simulink model "PI_VC_vs_UPI_CC_3ph_4w_v2023b"  (R2023b)
settings: Solver=FixedStepDiscrete  StartTime=0.0  StopTime=14  FixedStep=Ts_Power  MaxStep=1e-4  RelTol=1e-3
InitFcn:
  | run PI_VC_vs_UPI_CC_ini;
values from neighbouring files (symbols this model uses):
  C = 4e-6    (= 4e-06)    [PI_OL_vs_PI_CC_ini.m]    (also in PI_VC_vs_UPI_CC_ini.m)
  C_2 = 4e-6    (= 4e-06)    [PI_OL_vs_PI_CC_ini.m]    (also in PI_VC_vs_UPI_CC_ini.m)
  K_i_pll = 1.8/0.00251    (= 717.131474104)    [PI_OL_vs_PI_CC_ini.m]    (also in PI_VC_vs_UPI_CC_ini.m)
  K_p_pll = 1.8    [PI_OL_vs_PI_CC_ini.m]    (also in PI_VC_vs_UPI_CC_ini.m)
  Kp_i = 1*(L_t2 + L_s2)/tau_i    (= 2.5)    [PI_OL_vs_PI_CC_ini.m]    (also in PI_VC_vs_UPI_CC_ini.m)
  Kr_i = 2*(R_t2 + R_s2)/tau_i    (= 157.079632679)    [PI_OL_vs_PI_CC_ini.m]    (also in PI_VC_vs_UPI_CC_ini.m)
  L_line_12_13 = X_line_12_13/(2*pi*50)    (= 0.000798957814321)    [PI_OL_vs_PI_CC_ini.m]    (also in PI_VC_vs_UPI_CC_ini.m)
  L_line_13_14 = X_line_13_14/(2*pi*50)    (= 0.000200535228296)    [PI_OL_vs_PI_CC_ini.m]    (also in PI_VC_vs_UPI_CC_ini.m)
  L_n = L_t2 + L_s2    (= 0.0025)    [PI_OL_vs_PI_CC_ini.m]    (also in PI_VC_vs_UPI_CC_ini.m)
  L_s = 1.25e-3    (= 0.00125)    [PI_OL_vs_PI_CC_ini.m]    (also in PI_VC_vs_UPI_CC_ini.m)
  L_s2 = 1.25e-3    (= 0.00125)    [PI_OL_vs_PI_CC_ini.m]    (also in PI_VC_vs_UPI_CC_ini.m)
  L_t = 1.25e-3    (= 0.00125)    [PI_OL_vs_PI_CC_ini.m]    (also in PI_VC_vs_UPI_CC_ini.m)
  L_t2 = 1.25e-3    (= 0.00125)    [PI_OL_vs_PI_CC_ini.m]    (also in PI_VC_vs_UPI_CC_ini.m)
  omega = 2*pi*f    (= 314.159265359)    [PI_OL_vs_PI_CC_ini.m]    (also in PI_VC_vs_UPI_CC_ini.m)
  params_pi_cc = [S_b,U_b,K_p,T_p,K_q,T_q,X,R]    [PI_OL_vs_PI_CC_ini.m]    (also in PI_VC_vs_UPI_CC_ini.m)
  params_pi_vc = [S_b,U_b,K_p,T_p,K_q,T_q,Xv,Rv]    [PI_OL_vs_PI_CC_ini.m]    (also in PI_VC_vs_UPI_CC_ini.m)
  params_vc_cc = [R_t;L_t;R_s;L_s;K_pi;K_ii;C;K_pv;K_iv]    [PI_OL_vs_PI_CC_ini.m]    (also in PI_VC_vs_UPI_CC_ini.m)
  R_d = 10    [PI_OL_vs_PI_CC_ini.m]    (also in PI_VC_vs_UPI_CC_ini.m)
  R_d2 = 10    [PI_OL_vs_PI_CC_ini.m]    (also in PI_VC_vs_UPI_CC_ini.m)
  R_line_12_13 = (0.06)*Length    (= 0.24)    [PI_OL_vs_PI_CC_ini.m]    (also in PI_VC_vs_UPI_CC_ini.m)
  R_line_13_14 = (0.025)*Length    (= 0.1)    [PI_OL_vs_PI_CC_ini.m]    (also in PI_VC_vs_UPI_CC_ini.m)
  R_n = L_n*omega/10    (= 0.0785398163397)    [PI_OL_vs_PI_CC_ini.m]    (also in PI_VC_vs_UPI_CC_ini.m)
  R_s = L_s*omega/10    (= 0.0392699081699)    [PI_OL_vs_PI_CC_ini.m]    (also in PI_VC_vs_UPI_CC_ini.m)
  R_s2 = L_s*omega/10    (= 0.0392699081699)    [PI_OL_vs_PI_CC_ini.m]    (also in PI_VC_vs_UPI_CC_ini.m)
  R_t = L_t*omega/10    (= 0.0392699081699)    [PI_OL_vs_PI_CC_ini.m]    (also in PI_VC_vs_UPI_CC_ini.m)
  R_t2 = L_t*omega/10    (= 0.0392699081699)    [PI_OL_vs_PI_CC_ini.m]    (also in PI_VC_vs_UPI_CC_ini.m)
  S_b = 20e3    (= 20000)    [PI_OL_vs_PI_CC_ini.m]    (also in PI_VC_vs_UPI_CC_ini.m)
  Ts_Control = 50e-6    (= 5e-05)    [PI_OL_vs_PI_CC_ini.m]    (also in PI_VC_vs_UPI_CC_ini.m)
  Ts_Power = 50e-6    (= 5e-05)    [PI_OL_vs_PI_CC_ini.m]    (also in PI_VC_vs_UPI_CC_ini.m)
  v_dc = 800    [PI_OL_vs_PI_CC_ini.m]    (also in PI_VC_vs_UPI_CC_ini.m)
undefined symbols (not defined in the file or in its folder): DiscIntNeverNeededParam, omega_ref
libraries: spsFirstOrderFilterLib x32, spsUniversalBridgeLib x10, spsThreePhaseSeriesRLCBranchLib x9, spsPowerLib x6, spsThreePhaseVIMeasurementLib x6, eeGeneralControl x5, spsSeriesRLCLoadLib x5, spsRMSLib x4, spsSeriesRLCBranchLib x4, spsPower3phInstantaneousLib x3, spsThreePhaseBreakerLib x3, spsDCVoltageSourceLib x2
(part 2 of 3)

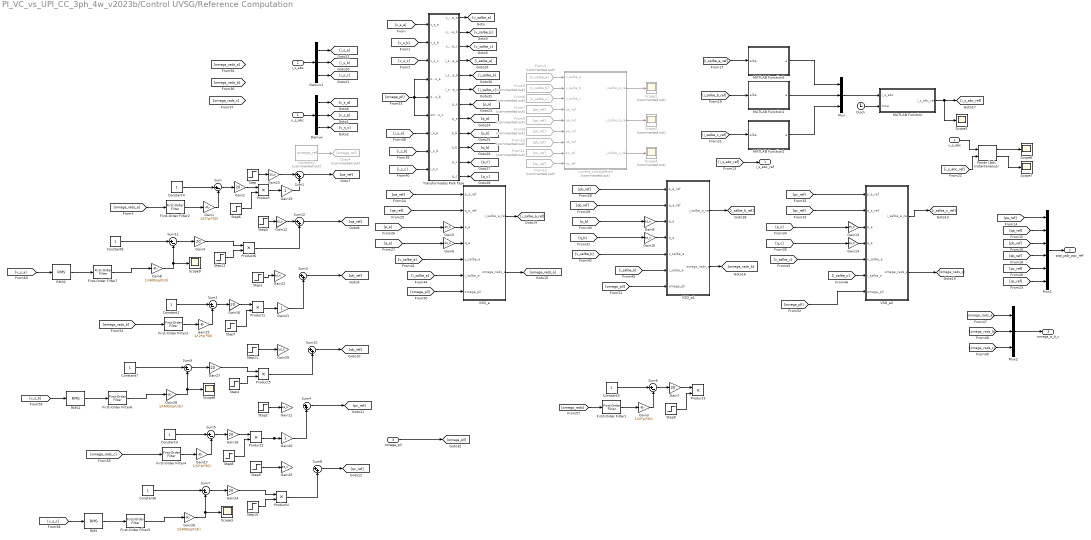
== system PI_VC_vs_UPI_CC_3ph_4w_v2023b/Control UVSG/Reference Computation ==
  v_s_abc : Inport
  i_s_abc : Inport  Port=2
  omega_pll : Inport  Port=3
  Clock : Clock
  Constant{1,3..8} (7 alike) : Constant
  Constant2 : Constant  Commented=on  Value=omega_ref
  Demux : Demux  Outputs=3
  Demux1 : Demux  Outputs=3
  First-Order Filter{1..7} (7 alike) : spsFirstOrderFilterLib/First-Order Filter  FilterType=Lowpass  Tc=10e-3  Ts=Ts_Control  Initialize=on  Vac_Init=[0, 0, 60]  Vdc_Init=0  PlotResponse=off  FreqRange="[0,  200,  1]"
  From10 : From  Commented=on  GotoTag=qb_ref
  From11 : From  Commented=on  GotoTag=pc_ref
  From12 : From  Commented=on  GotoTag=qc_ref
  From4 : From  Commented=on  GotoTag=v_salbe_a
  From5 : From  Commented=on  GotoTag=v_salbe_b
  From6 : From  Commented=on  GotoTag=v_salbe_c
  From7 : From  Commented=on  GotoTag=pa_ref
  From8 : From  Commented=on  GotoTag=pb_ref
  From9 : From  Commented=on  GotoTag=qa_ref
  Gain{1,3,15,17} (4 alike) : Gain  Gain=1/(2*pi*50)
  Gain{5..6,9..14,22..23,25,29} (12 alike) : Gain  Gain=3/S_b
  Gain{2,4,7,16,18,24,27} (7 alike) : Gain  Gain=20
  Gain19 : Gain
  Gain20 : Gain
  Gain21 : Gain
  Gain26 : Gain  Gain=1/(400/sqrt(3))
  Gain28 : Gain  Gain=1/(400/sqrt(3))
  Gain8 : Gain  Gain=1/(400/sqrt(3))
  Goto4 : Goto  Commented=on  GotoTag=omega_ref
  MATLAB Function : MATLAB Function  TreatAsAtomicUnit=on
  MATLAB Function1 : MATLAB Function  TreatAsAtomicUnit=on
  MATLAB Function2 : MATLAB Function  TreatAsAtomicUnit=on
  MATLAB Function5 : MATLAB Function  TreatAsAtomicUnit=on
  Mux : Mux  Inputs=3
  Mux1 : Mux  Inputs=6
  Mux2 : Mux  Inputs=3
  "Power (3ph, Instantaneous)" : spsPower3phInstantaneousLib/Power (3ph, Instantaneous)
  Product{,1..6} (7 alike) : Product
  RMS : spsRMSLib/RMS  TrueRMS=on  Freq=50  RMSInit=230  Ts=Ts_Control
  RMS1 : spsRMSLib/RMS  TrueRMS=on  Freq=50  RMSInit=230  Ts=Ts_Control
  RMS2 : spsRMSLib/RMS  TrueRMS=on  Freq=50  RMSInit=230  Ts=Ts_Control
  Scope1 : Scope  Commented=on
  Scope2 : Scope  Commented=on
  Scope{3,5..9} (6 alike) : Scope
  Scope4 : Scope  Commented=on
  Step : Step  Time=11  After=1000  SampleTime=0
  Step1 : Step  Time=6  After=1000  SampleTime=0
  Step{4,6..8,10,12} (6 alike) : Step  Time=7  SampleTime=0
  Step11 : Step  Time=0  After=0  SampleTime=0
  Step2 : Step  Time=6  After=1000  SampleTime=0
  Step3 : Step  Time=11  After=1000  SampleTime=0
  Step5 : Step  Time=0  After=0  SampleTime=0
  Step9 : Step  SampleTime=0
  Sum{,2,5..7,9,11} (7 alike) : Sum  Inputs=|+-
  Sum{1,3..4,8,10,12} (6 alike) : Sum  Inputs=|++
  Transformadas Park fase : Subsystem
  VSG_a : Subsystem
  VSG_a1 : Subsystem
  VSG_a2 : Subsystem
  current_computation : MATLAB Function  Commented=on  TreatAsAtomicUnit=on
  "v_s_abc " : InportShadow
  i_s_abc_ref : Outport  VectorParamsAs1DForOutWhenUnconnected=off
  pqa_pqb_pqc_ref : Outport  Port=2  VectorParamsAs1DForOutWhenUnconnected=off
  omega_a_b_c : Outport  Port=3  VectorParamsAs1DForOutWhenUnconnected=off
  wires:
  v_s_abc/1 -> Demux/1
  Demux/1 -> [v_s_a]
  Demux/2 -> [v_s_b]
  Demux/3 -> [v_s_c]
  Constant2/1 -> Goto4/1
  [v_s_a] -> Transformadas Park fase/1(v_s_a)
  [v_s_b] -> Transformadas Park fase/2(v_s_b)
  [v_s_c] -> Transformadas Park fase/3(v_s_c)
  Transformadas Park fase/1(v_salbe_a) -> [v_salbe_a]
  Transformadas Park fase/3(v_salbe_c) -> [v_salbe_c]
  Transformadas Park fase/2(v_salbe_b) -> [v_salbe_b]
  From4/1 -> current_computation/1(v_salbe_a)
  From5/1 -> current_computation/2(v_salbe_b)
  From6/1 -> current_computation/3(v_salbe_c)
  From7/1 -> current_computation/4(pa_ref)
  From9/1 -> current_computation/5(qa_ref)
  From8/1 -> current_computation/6(pb_ref)
  From10/1 -> current_computation/7(qb_ref)
  From11/1 -> current_computation/8(pc_ref)
  From12/1 -> current_computation/9(qc_ref)
  current_computation/1(i_salbe_a_ref) -> Scope1/1
  current_computation/2(i_salbe_b_ref) -> Scope2/1
  current_computation/3(i_salbe_c_ref) -> Scope4/1
  [i_salbe_b_ref] -> MATLAB Function1/1(albe)
  [i_salbe_c_ref] -> MATLAB Function2/1(albe)
  MATLAB Function5/1(a) -> Mux/1
  [i_s_abc_ref] -> "Power (3ph, Instantaneous)"/2
  "v_s_abc "/1 -> "Power (3ph, Instantaneous)"/1
  "Power (3ph, Instantaneous)"/1 -> Scope6/1
  "Power (3ph, Instantaneous)"/2 -> Scope7/1
  [i_s_abc_ref] -> i_s_abc_ref/1
  [i_salbe_a_ref] -> MATLAB Function5/1(albe)
  MATLAB Function1/1(a) -> Mux/2
  MATLAB Function2/1(a) -> Mux/3
  [pa_ref] -> Mux1/1
  [qa_ref] -> Mux1/2
  [pb_ref] -> Mux1/3
  [qb_ref] -> Mux1/4
  [pc_ref] -> Mux1/5
  [qc_ref] -> Mux1/6
  Mux1/1 -> pqa_pqb_pqc_ref/1
  VSG_a/2(omega_rads_a) -> [omega_rads_a]
  VSG_a1/2(omega_rads_a) -> [omega_rads_b]
  Demux1/3 -> [i_s_c]
  Demux1/2 -> [i_s_b]
  Demux1/1 -> [i_s_a]
  i_s_abc/1 -> Demux1/1
  [i_s_a] -> Transformadas Park fase/7(i_s_a)
  [i_s_b] -> Transformadas Park fase/8(i_s_b)
  [i_s_c] -> Transformadas Park fase/9(i_s_c)
  Transformadas Park fase/7(p_a) -> [p_a]
  Transformadas Park fase/8(q_a) -> [q_a]
  Transformadas Park fase/9(p_b) -> [p_b]
  Transformadas Park fase/10(q_b) -> [q_b]
  Transformadas Park fase/11(p_c) -> [p_c]
  Transformadas Park fase/12(q_c) -> [q_c]
  Transformadas Park fase/4(i_salbe_a) -> [i_salbe_a]
  Transformadas Park fase/5(i_salbe_b) -> [i_salbe_b]
  Transformadas Park fase/6(i_salbe_c) -> [i_salbe_c]
  VSG_a/1(i_salbe_a_ref) -> [i_salbe_a_ref]
  VSG_a1/1(i_salbe_a_ref) -> [i_salbe_b_ref]
  VSG_a2/1(i_salbe_a_ref) -> [i_salbe_c_ref]
  [pa_ref] -> VSG_a/1(p_a_ref)
  [qa_ref] -> VSG_a/2(q_a_ref)
  Gain5/1 -> VSG_a/3(p_a)
  Gain6/1 -> VSG_a/4(q_a)
  [pb_ref] -> VSG_a1/1(p_a_ref)
  [qb_ref] -> VSG_a1/2(q_a_ref)
  Gain9/1 -> VSG_a1/3(p_a)
  Gain10/1 -> VSG_a1/4(q_a)
  [qc_ref] -> VSG_a2/2(q_a_ref)
  Gain13/1 -> VSG_a2/3(p_a)
  Gain14/1 -> VSG_a2/4(q_a)
  [p_a] -> Gain5/1
  [q_a] -> Gain6/1
  [q_b] -> Gain10/1
  [p_c] -> Gain13/1
  [q_c] -> Gain14/1
  VSG_a2/2(omega_rads_a) -> [omega_rads_c]
  [v_salbe_a] -> VSG_a/5(v_salbe_a)
  [v_salbe_b] -> VSG_a1/5(v_salbe_a)
  [v_salbe_c] -> VSG_a2/5(v_salbe_a)
  [p_b] -> Gain9/1
  [i_salbe_a] -> VSG_a/6(i_salbe_a)
  [i_salbe_b] -> VSG_a1/6(i_salbe_a)
  [i_salbe_c] -> VSG_a2/6(i_salbe_a)
  Mux2/1 -> omega_a_b_c/1
  [omega_rads_a] -> Mux2/1
  [omega_rads_b] -> Mux2/2
  [omega_rads_c] -> Mux2/3
  omega_pll/1 -> [omega_pll]
  [omega_pll] -> VSG_a/7(omega_pll)
  [omega_pll] -> VSG_a1/7(omega_pll)
  [omega_pll] -> VSG_a2/7(omega_pll)
  Mux/1 -> MATLAB Function/1(i_s_abc)
  MATLAB Function/1(i_s_abc_ref) -> Scope5/1, [i_s_abc_ref]
  Clock/1 -> MATLAB Function/2(time)
  Gain2/1 -> Product/1
  [omega_rads_a] -> First-Order Filter2/1
  Step6/1 -> Product/2
  Gain1/1 -> Sum/2
  Constant4/1 -> Sum/1
  Sum/1 -> Gain2/1
  Product/1 -> Gain19/1
  Product1/1 -> Gain21/1
  Sum2/1 -> Gain16/1
  Constant1/1 -> Sum2/1
  Gain15/1 -> Sum2/2
  Step7/1 -> Product1/2
  [omega_rads_b] -> First-Order Filter3/1
  Gain16/1 -> Product1/1
  Gain18/1 -> Product2/1
  [omega_rads_c] -> First-Order Filter4/1
  Step8/1 -> Product2/2
  Gain17/1 -> Sum5/2
  Constant3/1 -> Sum5/1
  Sum5/1 -> Gain18/1
  Sum1/1 -> [pa_ref]
  Sum3/1 -> [pb_ref]
  Product2/1 -> Gain20/1
  Sum4/1 -> [pc_ref]
  Step2/1 -> Gain11/1
  Step1/1 -> Gain22/1
  Step/1 -> Gain23/1
  [pc_ref] -> VSG_a2/1(p_a_ref)
  [omega_pll] -> Transformadas Park fase/6(omega_rads_c), Transformadas Park fase/4(omega_rads_a), Transformadas Park fase/5(omega_rads_b)
  First-Order Filter1/1 -> Gain3/1
  [omega_rads] -> First-Order Filter1/1
  Step9/1 -> Product3/2
  Gain7/1 -> Product3/1
  Sum6/1 -> Gain7/1
  Gain3/1 -> Sum6/2
  Constant5/1 -> Sum6/1
  First-Order Filter2/1 -> Gain1/1
  First-Order Filter3/1 -> Gain15/1
  First-Order Filter4/1 -> Gain17/1
  Gain19/1 -> Sum1/2
  Gain21/1 -> Sum3/2
  Gain20/1 -> Sum4/2
  Gain23/1 -> Sum1/1
  Step5/1 -> Gain25/1
  Step10/1 -> Product4/2
  Gain24/1 -> Product4/1
  Sum7/1 -> Gain24/1
  Gain26/1 -> Scope3/1, Sum7/2
  [v_s_c] -> RMS/1
  Constant6/1 -> Sum7/1
  RMS/1 -> First-Order Filter5/1
  Sum8/1 -> [qc_ref]
  Product4/1 -> Sum8/2
  RMS1/1 -> First-Order Filter6/1
  Constant7/1 -> Sum9/1
  [v_s_b] -> RMS1/1
  Gain28/1 -> Sum9/2, Scope8/1
  Sum9/1 -> Gain27/1
  Gain27/1 -> Product5/1
  Step4/1 -> Product5/2
  Sum10/1 -> [qb_ref]
  Product5/1 -> Sum10/2
  Step11/1 -> Gain29/1
  Product6/1 -> Sum12/2
  Sum11/1 -> Gain4/1
  Gain4/1 -> Product6/1
  RMS2/1 -> First-Order Filter7/1
  [v_s_a] -> RMS2/1
  Gain8/1 -> Sum11/2, Scope9/1
  Step12/1 -> Product6/2
  Constant8/1 -> Sum11/1
  Gain12/1 -> Sum12/1
  Step3/1 -> Gain12/1
  Sum12/1 -> [qa_ref]
  First-Order Filter7/1 -> Gain8/1
  First-Order Filter6/1 -> Gain28/1
  First-Order Filter5/1 -> Gain26/1

== system PI_VC_vs_UPI_CC_3ph_4w_v2023b/Plant/Subsystem2 ==
  eta_abc : Inport
  eta_n : Inport  Port=2
  DC Voltage Source : spsDCVoltageSourceLib/DC Voltage Source  Amplitude=v_dc  Measurements=None
  Demux : Demux  Outputs=3
  Series RLC Branch : spsSeriesRLCBranchLib/Series RLC Branch  LConnTagsString=__new0  RConnTagsString=__new0  BranchType=RL  Resistance=R_n  Inductance=L_n  SetiL0=off  InitialCurrent=0  Capacitance=1e-6  Setx0=off  InitialVoltage=0  Measurements=None
  Three-Phase Series RLC Branch : spsThreePhaseSeriesRLCBranchLib/Three-Phase Series RLC Branch  LConnTagsString=A|B|C  RConnTagsString=A|B|C  BranchType=RL  Resistance=R_t  Inductance=L_t  Capacitance=1e-6  Measurements=None
  Three-Phase Series RLC Branch1 : spsThreePhaseSeriesRLCBranchLib/Three-Phase Series RLC Branch  LConnTagsString=A|B|C  RConnTagsString=A|B|C  BranchType=RL  Resistance=R_s  Inductance=L_s  Capacitance=1e-6  Measurements=None
  Three-Phase Series RLC Branch2 : spsThreePhaseSeriesRLCBranchLib/Three-Phase Series RLC Branch  LConnTagsString=A|B|C  RConnTagsString=A|B|C  BranchType=RC  Resistance=R_d  Inductance=L_t  Capacitance=C  Measurements=None
  Three-Phase V-I Measurement : spsThreePhaseVIMeasurementLib/Three-Phase V-I Measurement  VoltageMeasurement=phase-to-ground  SetLabelV=off  LabelV=Vabc  Vpu=off  VpuLL=off  CurrentMeasurement=yes  SetLabelI=off  LabelI=Iabc  Ipu=off  Pbase=100e6  Vbase=500e3  OutputType=Complex  PhasorSimulation=off  PSBequivalent=0
  Three-Phase V-I Measurement2 : spsThreePhaseVIMeasurementLib/Three-Phase V-I Measurement  VoltageMeasurement=phase-to-ground  SetLabelV=off  LabelV=Vabc  Vpu=off  VpuLL=off  CurrentMeasurement=no  SetLabelI=off  LabelI=Iabc  Ipu=off  Pbase=100e6  Vbase=500e3  OutputType=Complex  PhasorSimulation=off  PSBequivalent=0
  Universal Bridge : spsUniversalBridgeLib/Universal Bridge  Commented=on  Arms=3  SnubberResistance=1e5  SnubberCapacitance=inf  Device=Average-model based VSC  Ron=1e-3  Lon=0  ForwardVoltages="[  0  0  ]"  ForwardVoltage=0  GTOparameters=[ 10e-6 , 20e-6 ]  IGBTparameters=[ 1e-6 , 2e-6 ]  Measurements=None  Measurements_2=None  converterType=Rectifier
  Universal Bridge{1..2,4..5} (4 alike) : spsUniversalBridgeLib/Universal Bridge  Arms=1  SnubberResistance=1e5  SnubberCapacitance=inf  Device=Average-model based VSC  Ron=1e-3  Lon=0  ForwardVoltages="[  0  0  ]"  ForwardVoltage=0  GTOparameters=[ 10e-6 , 20e-6 ]  IGBTparameters=[ 1e-6 , 2e-6 ]  Measurements=None  Measurements_2=None  converterType=Rectifier
  Voltage Measurement : spsVoltageMeasurementLib/Voltage Measurement  PhasorSimulation=off  OutputType=Complex  PSBequivalent=0
  a : PMIOPort  Side=Right
  b : PMIOPort  Port=2  Side=Right
  c : PMIOPort  Port=3  Side=Right
  n : PMIOPort  Port=4  Side=Right
  v_cabc : Outport
  i_tabc : Outport  Port=2
  v_tabc : Outport  Port=3
  v_dc : Outport  Port=4
  wires:
  Three-Phase V-I Measurement/2 -> i_tabc/1
  Three-Phase V-I Measurement2/1 -> v_cabc/1
  Three-Phase V-I Measurement/1 -> v_tabc/1
  eta_abc/1 -> Demux/1
  Voltage Measurement/1 -> v_dc/1
  Demux/1 -> Universal Bridge2/1
  Demux/2 -> Universal Bridge4/1
  Demux/3 -> Universal Bridge5/1
  eta_n/1 -> Universal Bridge1/1
  connections:
  Three-Phase V-I Measurement/RConn3 -- Three-Phase Series RLC Branch/LConn3
  Three-Phase V-I Measurement/LConn2 -- Universal Bridge4/LConn1
  Three-Phase V-I Measurement/RConn1 -- Three-Phase Series RLC Branch/LConn1
  Three-Phase V-I Measurement2/LConn3 -- Three-Phase Series RLC Branch/RConn3 -- Three-Phase Series RLC Branch1/LConn3
  DC Voltage Source/RConn1 -- Universal Bridge1/RConn1 -- Universal Bridge5/RConn1 -- Universal Bridge4/RConn1 -- Universal Bridge2/RConn1 -- Voltage Measurement/LConn1
  DC Voltage Source/LConn1 -- Universal Bridge1/RConn2 -- Universal Bridge2/RConn2 -- Universal Bridge4/RConn2 -- Universal Bridge5/RConn2 -- Voltage Measurement/LConn2
  Three-Phase Series RLC Branch2/LConn2 -- Three-Phase V-I Measurement2/RConn2
  Three-Phase Series RLC Branch2/LConn1 -- Three-Phase V-I Measurement2/RConn3
  Three-Phase Series RLC Branch1/LConn2 -- Three-Phase V-I Measurement2/LConn2 -- Three-Phase Series RLC Branch/RConn2
  Three-Phase Series RLC Branch/LConn2 -- Three-Phase V-I Measurement/RConn2
  Three-Phase V-I Measurement/LConn1 -- Universal Bridge2/LConn1
  Three-Phase Series RLC Branch1/LConn1 -- Three-Phase V-I Measurement2/LConn1 -- Three-Phase Series RLC Branch/RConn1
  Three-Phase V-I Measurement2/RConn1 -- Three-Phase Series RLC Branch2/LConn3
  Three-Phase Series RLC Branch2/RConn3 -- n/RConn1 -- Series RLC Branch/RConn1 -- Three-Phase Series RLC Branch2/RConn1 -- Three-Phase Series RLC Branch2/RConn2
  Three-Phase V-I Measurement/LConn3 -- Universal Bridge5/LConn1
  a/RConn1 -- Three-Phase Series RLC Branch1/RConn1
  b/RConn1 -- Three-Phase Series RLC Branch1/RConn2
  Three-Phase Series RLC Branch1/RConn3 -- c/RConn1
  Universal Bridge1/LConn1 -- Series RLC Branch/LConn1

== system PI_VC_vs_UPI_CC_3ph_4w_v2023b/Plant/Subsystem3 ==
  eta_abc : Inport
  eta_n : Inport  Port=2
  DC Voltage Source : spsDCVoltageSourceLib/DC Voltage Source  Amplitude=v_dc  Measurements=None
  Demux : Demux  Outputs=3
  Series RLC Branch : spsSeriesRLCBranchLib/Series RLC Branch  LConnTagsString=__new0  RConnTagsString=__new0  BranchType=RL  Resistance=R_n  Inductance=L_n  SetiL0=off  InitialCurrent=0  Capacitance=1e-6  Setx0=off  InitialVoltage=0  Measurements=None
  Three-Phase Series RLC Branch : spsThreePhaseSeriesRLCBranchLib/Three-Phase Series RLC Branch  LConnTagsString=A|B|C  RConnTagsString=A|B|C  BranchType=RL  Resistance=R_t2  Inductance=L_t2  Capacitance=1e-6  Measurements=None
  Three-Phase Series RLC Branch1 : spsThreePhaseSeriesRLCBranchLib/Three-Phase Series RLC Branch  LConnTagsString=A|B|C  RConnTagsString=A|B|C  BranchType=RL  Resistance=R_s2  Inductance=L_s2  Capacitance=1e-6  Measurements=None
  Three-Phase Series RLC Branch2 : spsThreePhaseSeriesRLCBranchLib/Three-Phase Series RLC Branch  LConnTagsString=A|B|C  RConnTagsString=A|B|C  BranchType=RC  Resistance=R_d2  Inductance=L_t  Capacitance=C_2  Measurements=None
  Three-Phase V-I Measurement : spsThreePhaseVIMeasurementLib/Three-Phase V-I Measurement  VoltageMeasurement=phase-to-ground  SetLabelV=off  LabelV=Vabc  Vpu=off  VpuLL=off  CurrentMeasurement=yes  SetLabelI=off  LabelI=Iabc  Ipu=off  Pbase=100e6  Vbase=500e3  OutputType=Complex  PhasorSimulation=off  PSBequivalent=0
  Three-Phase V-I Measurement2 : spsThreePhaseVIMeasurementLib/Three-Phase V-I Measurement  VoltageMeasurement=phase-to-ground  SetLabelV=off  LabelV=Vabc  Vpu=off  VpuLL=off  CurrentMeasurement=no  SetLabelI=off  LabelI=Iabc  Ipu=off  Pbase=100e6  Vbase=500e3  OutputType=Complex  PhasorSimulation=off  PSBequivalent=0
  Universal Bridge : spsUniversalBridgeLib/Universal Bridge  Commented=on  Arms=3  SnubberResistance=1e5  SnubberCapacitance=inf  Device=Average-model based VSC  Ron=1e-3  Lon=0  ForwardVoltages="[  0  0  ]"  ForwardVoltage=0  GTOparameters=[ 10e-6 , 20e-6 ]  IGBTparameters=[ 1e-6 , 2e-6 ]  Measurements=None  Measurements_2=None  converterType=Rectifier
  Universal Bridge{1..2,4..5} (4 alike) : spsUniversalBridgeLib/Universal Bridge  Arms=1  SnubberResistance=1e5  SnubberCapacitance=inf  Device=Average-model based VSC  Ron=1e-3  Lon=0  ForwardVoltages="[  0  0  ]"  ForwardVoltage=0  GTOparameters=[ 10e-6 , 20e-6 ]  IGBTparameters=[ 1e-6 , 2e-6 ]  Measurements=None  Measurements_2=None  converterType=Rectifier
  Voltage Measurement : spsVoltageMeasurementLib/Voltage Measurement  PhasorSimulation=off  OutputType=Complex  PSBequivalent=0
  a : PMIOPort  Side=Right
  b : PMIOPort  Port=2  Side=Right
  c : PMIOPort  Port=3  Side=Right
  n : PMIOPort  Port=4  Side=Right
  v_cabc : Outport
  i_tabc : Outport  Port=2
  v_tabc : Outport  Port=3
  v_dc : Outport  Port=4
  wires:
  eta_n/1 -> Universal Bridge1/1
  Demux/3 -> Universal Bridge5/1
  Demux/2 -> Universal Bridge4/1
  Demux/1 -> Universal Bridge2/1
  Voltage Measurement/1 -> v_dc/1
  eta_abc/1 -> Demux/1
  Three-Phase V-I Measurement/1 -> v_tabc/1
  Three-Phase V-I Measurement2/1 -> v_cabc/1
  Three-Phase V-I Measurement/2 -> i_tabc/1
  connections:
  Universal Bridge1/LConn1 -- Series RLC Branch/LConn1
  Three-Phase Series RLC Branch1/RConn3 -- c/RConn1
  b/RConn1 -- Three-Phase Series RLC Branch1/RConn2
  a/RConn1 -- Three-Phase Series RLC Branch1/RConn1
  Three-Phase V-I Measurement/LConn3 -- Universal Bridge5/LConn1
  n/RConn1 -- Three-Phase Series RLC Branch2/RConn2 -- Three-Phase Series RLC Branch2/RConn1 -- Series RLC Branch/RConn1 -- Three-Phase Series RLC Branch2/RConn3
  Three-Phase V-I Measurement2/RConn1 -- Three-Phase Series RLC Branch2/LConn3
  Three-Phase Series RLC Branch/RConn1 -- Three-Phase V-I Measurement2/LConn1 -- Three-Phase Series RLC Branch1/LConn1
  Three-Phase V-I Measurement/LConn1 -- Universal Bridge2/LConn1
  Three-Phase Series RLC Branch/LConn2 -- Three-Phase V-I Measurement/RConn2
  Three-Phase Series RLC Branch/RConn2 -- Three-Phase V-I Measurement2/LConn2 -- Three-Phase Series RLC Branch1/LConn2
  Three-Phase Series RLC Branch2/LConn1 -- Three-Phase V-I Measurement2/RConn3
  Three-Phase Series RLC Branch2/LConn2 -- Three-Phase V-I Measurement2/RConn2
  Universal Bridge1/RConn2 -- Universal Bridge5/RConn2 -- Universal Bridge4/RConn2 -- Universal Bridge2/RConn2 -- Voltage Measurement/LConn2 -- DC Voltage Source/LConn1
  Universal Bridge1/RConn1 -- Universal Bridge5/RConn1 -- Universal Bridge4/RConn1 -- Voltage Measurement/LConn1 -- DC Voltage Source/RConn1 -- Universal Bridge2/RConn1
  Three-Phase Series RLC Branch1/LConn3 -- Three-Phase Series RLC Branch/RConn3 -- Three-Phase V-I Measurement2/LConn3
  Three-Phase V-I Measurement/RConn1 -- Three-Phase Series RLC Branch/LConn1
  Three-Phase V-I Measurement/LConn2 -- Universal Bridge4/LConn1
  Three-Phase V-I Measurement/RConn3 -- Three-Phase Series RLC Branch/LConn3

== system PI_VC_vs_UPI_CC_3ph_4w_v2023b/Control UVSG/Control corriente en alpha-beta/Resonant Controller. Double Integrator ==
  i_sal_ref : Inport
  i_sal : Inport  Port=2
  Vdc : Inport  Port=3
  i_sbe_ref : Inport  Port=4
  i_sbe : Inport  Port=5
  omega_PLL : Inport  Port=6
  v_sal : Inport  Port=7
  v_sbe : Inport  Port=8
  Divide : Product  Inputs=*/
  Divide1 : Product  Inputs=*/
  Gain1 : Gain  Gain=Kp_i
  Gain10 : Gain  Gain=2
  Gain7 : Gain  Gain=2
  Gain8 : Gain  Gain=Kp_i
  Mux : Mux  Inputs=2
  Scope7 : Scope
  Subsystem1 : Subsystem
  Subsystem2 : Subsystem
  Sum{4..6,13} (4 alike) : Sum  Inputs=|++
  Sum7 : Sum  Inputs=|+-
  Sum9 : Sum  Inputs=|+-
  omega_PLL_1 : InportShadow  Port=6
  eta_albe : Outport
  wires:
  Gain1/1 -> Sum6/1
  Gain8/1 -> Sum13/1
  i_sbe_ref/1 -> Sum9/1
  omega_PLL_1/1 -> Subsystem1/2(omega_PLL)
  i_sal_ref/1 -> Sum7/1
  Sum13/1 -> Sum4/1
  Vdc/1 -> Divide/2, Divide1/2
  Sum5/1 -> Gain10/1
  Sum7/1 -> Subsystem1/1(error), Gain8/1, Scope7/1
  Sum6/1 -> Sum5/1
  Sum4/1 -> Gain7/1
  Divide1/1 -> Mux/2
  Divide/1 -> Mux/1
  Gain7/1 -> Divide/1
  Subsystem1/1(out) -> Sum13/2
  Sum9/1 -> Subsystem2/1(error), Gain1/1
  Subsystem2/1(out) -> Sum6/2
  v_sal/1 -> Sum4/2
  Gain10/1 -> Divide1/1
  omega_PLL/1 -> Subsystem2/2(omega_PLL)
  Mux/1 -> eta_albe/1
  i_sal/1 -> Sum7/2
  i_sbe/1 -> Sum9/2
  v_sbe/1 -> Sum5/2

== system PI_VC_vs_UPI_CC_3ph_4w_v2023b/Control UVSG/Control corriente en alpha-beta/Resonant Controller. Impulse invariant ==
  i_sal_ref : Inport
  i_sal : Inport  Port=2
  Vdc : Inport  Port=3
  i_sbe_ref : Inport  Port=4
  i_sbe : Inport  Port=5
  omega_PLL : Inport  Port=6
  v_sal : Inport  Port=7
  v_sbe : Inport  Port=8
  Divide : Product  Inputs=*/
  Divide1 : Product  Inputs=*/
  Gain1 : Gain  Gain=Kp_i
  Gain10 : Gain  Gain=2
  Gain7 : Gain  Gain=2
  Gain8 : Gain  Gain=Kp_i
  Mux : Mux  Inputs=2
  Scope7 : Scope
  Subsystem : Subsystem
  Subsystem1 : Subsystem
  Sum{4..6,13} (4 alike) : Sum  Inputs=|++
  Sum7 : Sum  Inputs=|+-
  Sum9 : Sum  Inputs=|+-
  omega_PLL_1 : InportShadow  Port=6
  eta_albe : Outport
  wires:
  Gain1/1 -> Sum6/1
  Gain8/1 -> Sum13/1
  i_sbe_ref/1 -> Sum9/1
  i_sal_ref/1 -> Sum7/1
  Sum13/1 -> Sum4/1
  Vdc/1 -> Divide/2, Divide1/2
  Sum5/1 -> Gain10/1
  Sum7/1 -> Subsystem1/1(error), Gain8/1, Scope7/1
  Sum6/1 -> Sum5/1
  Sum4/1 -> Gain7/1
  Divide1/1 -> Mux/2
  Divide/1 -> Mux/1
  Gain7/1 -> Divide/1
  Sum9/1 -> Subsystem/1(error), Gain1/1
  v_sal/1 -> Sum4/2
  Gain10/1 -> Divide1/1
  Mux/1 -> eta_albe/1
  i_sal/1 -> Sum7/2
  i_sbe/1 -> Sum9/2
  v_sbe/1 -> Sum5/2
  omega_PLL/1 -> Subsystem/2(omega_PLL)
  omega_PLL_1/1 -> Subsystem1/2(omega_PLL)
  Subsystem1/1(y) -> Sum13/2
  Subsystem/1(y) -> Sum6/2

== system PI_VC_vs_UPI_CC_3ph_4w_v2023b/Control UVSG/Control corriente en alpha-beta/Subsystem ==
  In1 : Inport
  Demux : Demux  Outputs=2
  Mux : Mux  Inputs=2
  Unit Delay1 : UnitDelay  SampleTime=Ts_Control  HasFrameUpgradeWarning=on
  Unit Delay2 : UnitDelay  SampleTime=Ts_Control  HasFrameUpgradeWarning=on
  Out1 : Outport
  wires:
  In1/1 -> Demux/1
  Demux/1 -> Unit Delay2/1
  Demux/2 -> Unit Delay1/1
  Mux/1 -> Out1/1
  Unit Delay2/1 -> Mux/1
  Unit Delay1/1 -> Mux/2

== system PI_VC_vs_UPI_CC_3ph_4w_v2023b/Control UVSG/Control corriente en alpha-beta/Subsystem1 ==
  In1 : Inport
  Demux : Demux  Outputs=2
  Mux : Mux  Inputs=2
  Unit Delay1 : UnitDelay  SampleTime=Ts_Control  HasFrameUpgradeWarning=on
  Unit Delay2 : UnitDelay  SampleTime=Ts_Control  HasFrameUpgradeWarning=on
  u_aux_1 : Outport
  wires:
  Unit Delay1/1 -> Mux/2
  Unit Delay2/1 -> Mux/1
  Mux/1 -> u_aux_1/1
  Demux/2 -> Unit Delay1/1
  Demux/1 -> Unit Delay2/1
  In1/1 -> Demux/1

== system PI_VC_vs_UPI_CC_3ph_4w_v2023b/Control UVSG/Control corriente en alpha-beta/Subsystem2 ==
  In1 : Inport
  Demux : Demux  Outputs=2
  Mux : Mux  Inputs=2
  Unit Delay1 : UnitDelay  SampleTime=Ts_Control  HasFrameUpgradeWarning=on
  Unit Delay2 : UnitDelay  SampleTime=Ts_Control  HasFrameUpgradeWarning=on
  Out1 : Outport
  wires:
  In1/1 -> Demux/1
  Demux/1 -> Unit Delay2/1
  Demux/2 -> Unit Delay1/1
  Mux/1 -> Out1/1
  Unit Delay2/1 -> Mux/1
  Unit Delay1/1 -> Mux/2

== system PI_VC_vs_UPI_CC_3ph_4w_v2023b/Control UVSG/Control corriente en alpha-beta/Subsystem3 ==
  In1 : Inport
  Demux : Demux  Outputs=2
  Mux : Mux  Inputs=2
  Unit Delay1 : UnitDelay  SampleTime=Ts_Control  HasFrameUpgradeWarning=on
  Unit Delay2 : UnitDelay  SampleTime=Ts_Control  HasFrameUpgradeWarning=on
  Out1 : Outport
  wires:
  Unit Delay1/1 -> Mux/2
  Unit Delay2/1 -> Mux/1
  Mux/1 -> Out1/1
  Demux/2 -> Unit Delay1/1
  Demux/1 -> Unit Delay2/1
  In1/1 -> Demux/1

== system PI_VC_vs_UPI_CC_3ph_4w_v2023b/Control UVSG/Control corriente en alpha-beta/Subsystem4 ==
  In1 : Inport
  Demux : Demux  Outputs=2
  Mux : Mux  Inputs=2
  Unit Delay1 : UnitDelay  SampleTime=Ts_Control  HasFrameUpgradeWarning=on
  Unit Delay2 : UnitDelay  SampleTime=Ts_Control  HasFrameUpgradeWarning=on
  Out1 : Outport
  wires:
  In1/1 -> Demux/1
  Demux/1 -> Unit Delay2/1
  Demux/2 -> Unit Delay1/1
  Mux/1 -> Out1/1
  Unit Delay2/1 -> Mux/1
  Unit Delay1/1 -> Mux/2

== system PI_VC_vs_UPI_CC_3ph_4w_v2023b/Control UVSG/Control corriente en alpha-beta/Subsystem5 ==
  In1 : Inport
  Demux : Demux  Outputs=2
  Mux : Mux  Inputs=2
  Unit Delay1 : UnitDelay  SampleTime=Ts_Control  HasFrameUpgradeWarning=on
  Unit Delay2 : UnitDelay  SampleTime=Ts_Control  HasFrameUpgradeWarning=on
  y_aux_2 : Outport
  wires:
  Unit Delay1/1 -> Mux/2
  Unit Delay2/1 -> Mux/1
  Mux/1 -> y_aux_2/1
  Demux/2 -> Unit Delay1/1
  Demux/1 -> Unit Delay2/1
  In1/1 -> Demux/1

== system PI_VC_vs_UPI_CC_3ph_4w_v2023b/Control UVSG/PARK_PLL/PLL ==
  v_sabc : Inport
  Demux : Demux  Outputs=2
  Discrete-Time Integrator1 : DiscreteIntegrator  InitialCondition=2*pi*50  SampleTime=Ts_Control  ICPrevOutput=DiscIntNeverNeededParam  ICPrevScaledInput=DiscIntNeverNeededParam
  Integrator with Wrapped State (Discrete or Continuous) : eeGeneralControl/Integrator with Wrapped State (Discrete or Continuous)  LabelModeActiveChoice=Discrete  WrappedStateUpperValue=2*pi  WrappedStateLowerValue=0  x0=0  Ts=Ts_Control
  Ki : Gain  Gain=K_i_pll
  Kp : Gain  Gain=K_p_pll
  MATLAB Function1 : MATLAB Function  TreatAsAtomicUnit=on
  Sum : Sum  Inputs=|++
  omega : Outport  VectorParamsAs1DForOutWhenUnconnected=off
  theta : Outport  Port=2  VectorParamsAs1DForOutWhenUnconnected=off
  wires:
  MATLAB Function1/1(dq) -> Demux/1
  v_sabc/1 -> MATLAB Function1/2(abc)
  [theta] -> MATLAB Function1/1(theta)
  Ki/1 -> Discrete-Time Integrator1/1
  Kp/1 -> Sum/1
  Discrete-Time Integrator1/1 -> Sum/2
  Sum/1 -> Integrator with Wrapped State (Discrete or Continuous)/1, omega/1
  Integrator with Wrapped State (Discrete or Continuous)/1 -> [theta], theta/1
  Demux/1 -> Ki/1, Kp/1

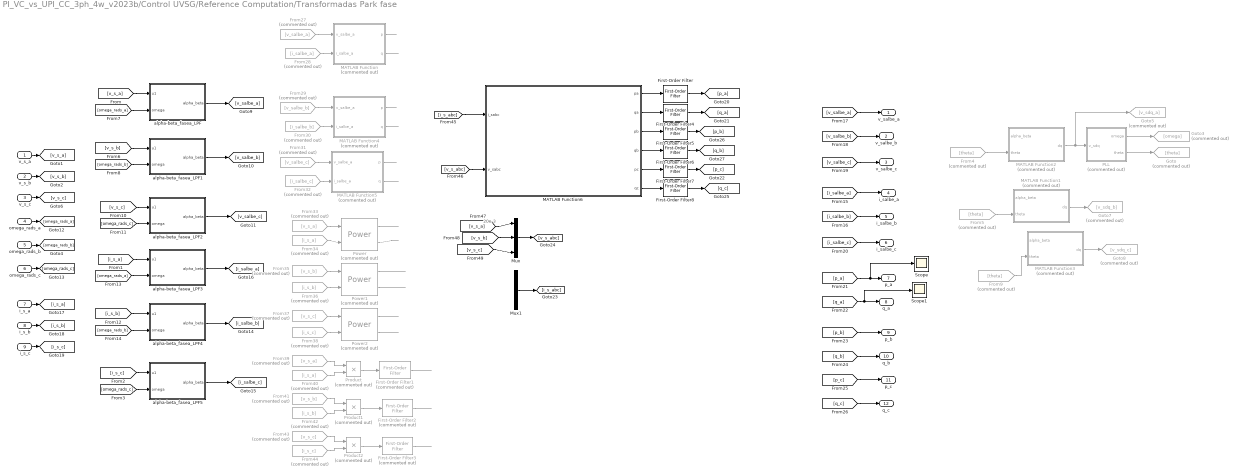
== system PI_VC_vs_UPI_CC_3ph_4w_v2023b/Control UVSG/Reference Computation/Transformadas Park fase ==
  note: 20e-3
  v_s_a : Inport
  v_s_b : Inport  Port=2
  v_s_c : Inport  Port=3
  omega_rads_a : Inport  Port=4
  omega_rads_b : Inport  Port=5
  omega_rads_c : Inport  Port=6
  i_s_a : Inport  Port=7
  i_s_b : Inport  Port=8
  i_s_c : Inport  Port=9
  First-Order Filter{,4..8} (6 alike) : spsFirstOrderFilterLib/First-Order Filter  FilterType=Lowpass  Tc=20e-3  Ts=Ts_Control  Initialize=on  Vac_Init=[0, 0, 60]  Vdc_Init=0  PlotResponse=off  FreqRange="[0,  200,  1]"
  First-Order Filter1 : spsFirstOrderFilterLib/First-Order Filter  Commented=on  FilterType=Lowpass  Tc=20e-3  Ts=Ts_Control  Initialize=on  Vac_Init=[0, 0, 60]  Vdc_Init=0  PlotResponse=off  FreqRange="[0,  200,  1]"
  First-Order Filter2 : spsFirstOrderFilterLib/First-Order Filter  Commented=on  FilterType=Lowpass  Tc=20e-3  Ts=Ts_Control  Initialize=on  Vac_Init=[0, 0, 60]  Vdc_Init=0  PlotResponse=off  FreqRange="[0,  200,  1]"
  First-Order Filter3 : spsFirstOrderFilterLib/First-Order Filter  Commented=on  FilterType=Lowpass  Tc=20e-3  Ts=Ts_Control  Initialize=on  Vac_Init=[0, 0, 60]  Vdc_Init=0  PlotResponse=off  FreqRange="[0,  200,  1]"
  From27 : From  Commented=on  GotoTag=v_salbe_a
  From28 : From  Commented=on  GotoTag=i_salbe_a
  From29 : From  Commented=on  GotoTag=v_salbe_b
  From30 : From  Commented=on  GotoTag=i_salbe_b
  From31 : From  Commented=on  GotoTag=v_salbe_c
  From32 : From  Commented=on  GotoTag=i_salbe_c
  From33 : From  Commented=on  GotoTag=v_s_a
  From34 : From  Commented=on  GotoTag=i_s_a
  From35 : From  Commented=on  GotoTag=v_s_b
  From36 : From  Commented=on  GotoTag=i_s_b
  From37 : From  Commented=on  GotoTag=v_s_c
  From38 : From  Commented=on  GotoTag=i_s_c
  From39 : From  Commented=on  GotoTag=v_s_a
  From4 : From  Commented=on  GotoTag=theta
  From40 : From  Commented=on  GotoTag=i_s_a
  From41 : From  Commented=on  GotoTag=v_s_b
  From42 : From  Commented=on  GotoTag=i_s_b
  From43 : From  Commented=on  GotoTag=v_s_c
  From44 : From  Commented=on  GotoTag=i_s_c
  From5 : From  Commented=on  GotoTag=theta
  From9 : From  Commented=on  GotoTag=theta
  Goto : Goto  Commented=on  GotoTag=theta
  Goto3 : Goto  Commented=on  GotoTag=omega
  Goto5 : Goto  Commented=on  GotoTag=v_sdq_a
  Goto7 : Goto  Commented=on  GotoTag=v_sdq_b
  Goto8 : Goto  Commented=on  GotoTag=v_sdq_c
  MATLAB Function : MATLAB Function  Commented=on  TreatAsAtomicUnit=on
  MATLAB Function1 : MATLAB Function  Commented=on  TreatAsAtomicUnit=on
  MATLAB Function2 : MATLAB Function  Commented=on  TreatAsAtomicUnit=on
  MATLAB Function3 : MATLAB Function  Commented=on  TreatAsAtomicUnit=on
  MATLAB Function4 : MATLAB Function  Commented=on  TreatAsAtomicUnit=on
  MATLAB Function5 : MATLAB Function  Commented=on  TreatAsAtomicUnit=on
  MATLAB Function6 : MATLAB Function  TreatAsAtomicUnit=on
  Mux : Mux  Inputs=3
  Mux1 : Mux  Inputs=3
  PLL : Subsystem  Commented=on
  Power : spsPowerLib/Power  Commented=on  Freq=50  Vinit=[1, 0]  Iinit=[1, 0]  Ts=Ts_Control
  Power1 : spsPowerLib/Power  Commented=on  Freq=50  Vinit=[1, 0]  Iinit=[1, 0]  Ts=Ts_Control
  Power2 : spsPowerLib/Power  Commented=on  Freq=50  Vinit=[1, 0]  Iinit=[1, 0]  Ts=Ts_Control
  Product : Product  Commented=on
  Product1 : Product  Commented=on
  Product2 : Product  Commented=on
  Scope : Scope
  Scope1 : Scope
  alpha-beta_fasea_LPF : Subsystem
  alpha-beta_fasea_LPF1 : Subsystem
  alpha-beta_fasea_LPF2 : Subsystem
  alpha-beta_fasea_LPF3 : Subsystem
  alpha-beta_fasea_LPF4 : Subsystem
  alpha-beta_fasea_LPF5 : Subsystem
  v_salbe_a : Outport  VectorParamsAs1DForOutWhenUnconnected=off
  v_salbe_b : Outport  Port=2  VectorParamsAs1DForOutWhenUnconnected=off
  v_salbe_c : Outport  Port=3  VectorParamsAs1DForOutWhenUnconnected=off
  i_salbe_a : Outport  Port=4  VectorParamsAs1DForOutWhenUnconnected=off
  i_salbe_b : Outport  Port=5  VectorParamsAs1DForOutWhenUnconnected=off
  i_salbe_c : Outport  Port=6  VectorParamsAs1DForOutWhenUnconnected=off
  p_a : Outport  Port=7  VectorParamsAs1DForOutWhenUnconnected=off
  q_a : Outport  Port=8  VectorParamsAs1DForOutWhenUnconnected=off
  p_b : Outport  Port=9  VectorParamsAs1DForOutWhenUnconnected=off
  q_b : Outport  Port=10  VectorParamsAs1DForOutWhenUnconnected=off
  p_c : Outport  Port=11  VectorParamsAs1DForOutWhenUnconnected=off
  q_c : Outport  Port=12  VectorParamsAs1DForOutWhenUnconnected=off
  wires:
  PLL/2(theta) -> Goto/1
  MATLAB Function1/1(dq) -> Goto7/1
  [v_s_b] -> alpha-beta_fasea_LPF1/1(u1)
  MATLAB Function2/1(dq) -> Goto5/1, PLL/1(v_sdq)
  [v_s_a] -> alpha-beta_fasea_LPF/1(u1)
  [omega_rads_c] -> alpha-beta_fasea_LPF2/2(omega)
  MATLAB Function3/1(dq) -> Goto8/1
  [omega_rads_a] -> alpha-beta_fasea_LPF/2(omega)
  PLL/1(omega) -> Goto3/1
  alpha-beta_fasea_LPF/1(alpha_beta) -> [v_salbe_a]
  From5/1 -> MATLAB Function1/2(theta)
  alpha-beta_fasea_LPF2/1(alpha_beta) -> [v_salbe_c]
  From4/1 -> MATLAB Function2/2(theta)
  [v_s_c] -> alpha-beta_fasea_LPF2/1(u1)
  [omega_rads_b] -> alpha-beta_fasea_LPF1/2(omega)
  alpha-beta_fasea_LPF1/1(alpha_beta) -> [v_salbe_b]
  From9/1 -> MATLAB Function3/2(theta)
  v_s_a/1 -> [v_s_a]
  v_s_b/1 -> [v_s_b]
  v_s_c/1 -> [v_s_c]
  omega_rads_a/1 -> [omega_rads_a]
  [v_salbe_a] -> v_salbe_a/1
  [v_salbe_b] -> v_salbe_b/1
  [v_salbe_c] -> v_salbe_c/1
  omega_rads_b/1 -> [omega_rads_b]
  omega_rads_c/1 -> [omega_rads_c]
  alpha-beta_fasea_LPF4/1(alpha_beta) -> [i_salbe_b]
  [omega_rads_b] -> alpha-beta_fasea_LPF4/2(omega)
  [i_s_c] -> alpha-beta_fasea_LPF5/1(u1)
  alpha-beta_fasea_LPF5/1(alpha_beta) -> [i_salbe_c]
  alpha-beta_fasea_LPF3/1(alpha_beta) -> [i_salbe_a]
  [omega_rads_a] -> alpha-beta_fasea_LPF3/2(omega)
  [omega_rads_c] -> alpha-beta_fasea_LPF5/2(omega)
  [i_s_a] -> alpha-beta_fasea_LPF3/1(u1)
  [i_s_b] -> alpha-beta_fasea_LPF4/1(u1)
  [i_salbe_c] -> i_salbe_c/1
  [i_salbe_b] -> i_salbe_b/1
  [i_salbe_a] -> i_salbe_a/1
  [p_a] -> Scope/1, p_a/1
  [q_a] -> Scope1/1, q_a/1
  [q_b] -> q_b/1
  [p_b] -> p_b/1
  [p_c] -> p_c/1
  [q_c] -> q_c/1
  i_s_c/1 -> [i_s_c]
  i_s_b/1 -> [i_s_b]
  i_s_a/1 -> [i_s_a]
  From27/1 -> MATLAB Function/1(v_salbe_a)
  From28/1 -> MATLAB Function/2(i_salbe_a)
  MATLAB Function/1(p) -> ?
  MATLAB Function/2(q) -> ?
  MATLAB Function4/2(q) -> ?
  MATLAB Function4/1(p) -> ?
  From30/1 -> MATLAB Function4/2(i_salbe_a)
  From29/1 -> MATLAB Function4/1(v_salbe_a)
  From31/1 -> MATLAB Function5/1(v_salbe_a)
  From32/1 -> MATLAB Function5/2(i_salbe_a)
  MATLAB Function5/1(p) -> ?
  MATLAB Function5/2(q) -> ?
  From33/1 -> Power/1
  From34/1 -> Power/2
  Power/1 -> ?
  Power/2 -> ?
  Power1/2 -> ?
  Power1/1 -> ?
  From36/1 -> Power1/2
  From35/1 -> Power1/1
  From37/1 -> Power2/1
  From38/1 -> Power2/2
  Power2/1 -> ?
  Power2/2 -> ?
  From39/1 -> Product/1
  From40/1 -> Product/2
  From42/1 -> Product1/2
  From41/1 -> Product1/1
  From43/1 -> Product2/1
  From44/1 -> Product2/2
  Product2/1 -> First-Order Filter3/1
  Product1/1 -> First-Order Filter2/1
  Product/1 -> First-Order Filter1/1
  First-Order Filter1/1 -> ?
  First-Order Filter2/1 -> ?
  First-Order Filter3/1 -> ?
  MATLAB Function6/1(pa) -> First-Order Filter/1
  MATLAB Function6/3(pb) -> First-Order Filter5/1
  MATLAB Function6/2(qa) -> First-Order Filter4/1
  MATLAB Function6/4(qb) -> First-Order Filter6/1
  [v_s_abc] -> MATLAB Function6/2(v_sabc)
  MATLAB Function6/5(pc) -> First-Order Filter7/1
  [i_s_abc] -> MATLAB Function6/1(i_sabc)
  MATLAB Function6/6(qc) -> First-Order Filter8/1
  First-Order Filter/1 -> [p_a]
  First-Order Filter4/1 -> [q_a]
  First-Order Filter5/1 -> [p_b]
  First-Order Filter6/1 -> [q_b]
  First-Order Filter7/1 -> [p_c]
  First-Order Filter8/1 -> [q_c]
  Mux/1 -> [v_s_abc]
  [v_s_a] -> Mux/1
  [v_s_b] -> Mux/2
  [v_s_c] -> Mux/3
  Mux1/1 -> [i_s_abc]

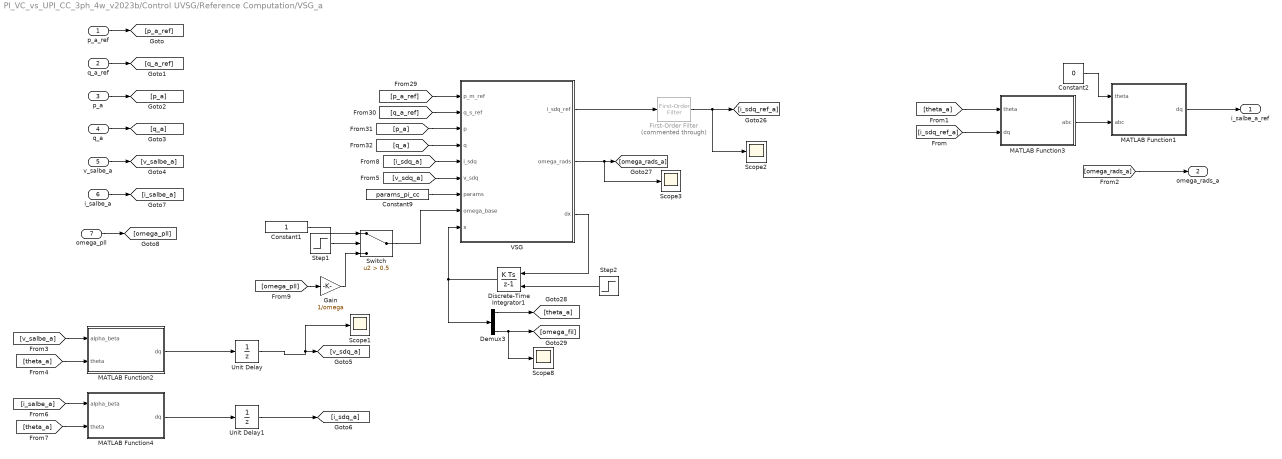
== system PI_VC_vs_UPI_CC_3ph_4w_v2023b/Control UVSG/Reference Computation/VSG_a ==
  p_a_ref : Inport
  q_a_ref : Inport  Port=2
  p_a : Inport  Port=3
  q_a : Inport  Port=4
  v_salbe_a : Inport  Port=5
  i_salbe_a : Inport  Port=6
  omega_pll : Inport  Port=7
  Constant1 : Constant
  Constant2 : Constant  Value=0
  Constant9 : Constant  Value=params_pi_cc
  Demux3 : Demux
  Discrete-Time Integrator1 : DiscreteIntegrator  ExternalReset=rising  InitialCondition=[0;0;0;2*pi*50]  SampleTime=Ts_Control  ICPrevOutput=DiscIntNeverNeededParam  ICPrevScaledInput=DiscIntNeverNeededParam
  First-Order Filter : spsFirstOrderFilterLib/First-Order Filter  Commented=through  FilterType=Lowpass  Tc=2.4e-3  Ts=Ts_Control  Initialize=on  Vac_Init=[0, 0, 60]  Vdc_Init=0  PlotResponse=off  FreqRange="[0,  200,  1]"
  Gain : Gain  Gain=1/omega
  MATLAB Function1 : MATLAB Function  TreatAsAtomicUnit=on
  MATLAB Function2 : MATLAB Function  TreatAsAtomicUnit=on
  MATLAB Function3 : MATLAB Function  TreatAsAtomicUnit=on
  MATLAB Function4 : MATLAB Function  TreatAsAtomicUnit=on
  Scope{1..3,8} (4 alike) : Scope
  Step1 : Step  SampleTime=0
  Step2 : Step  Time=0  SampleTime=0
  Switch : Switch  Criteria=u2 > Threshold  Threshold=0.5  SaturateOnIntegerOverflow=off  InputSameDT=off
  Unit Delay : UnitDelay  SampleTime=-1  HasFrameUpgradeWarning=on
  Unit Delay1 : UnitDelay  SampleTime=-1  HasFrameUpgradeWarning=on
  VSG : MATLAB Function  TreatAsAtomicUnit=on
  i_salbe_a_ref : Outport  VectorParamsAs1DForOutWhenUnconnected=off
  omega_rads_a : Outport  Port=2  VectorParamsAs1DForOutWhenUnconnected=off
  wires:
  [p_a_ref] -> VSG/1(p_m_ref)
  [q_a] -> VSG/4(q)
  Constant9/1 -> VSG/7(params)
  Demux3/4 -> Scope8/1, [omega_fil]
  Demux3/1 -> [theta_a]
  VSG/1(i_sdq_ref) -> First-Order Filter/1
  Discrete-Time Integrator1/1 -> Demux3/1, VSG/9(x)
  VSG/2(omega_rads) -> Scope3/1, [omega_rads_a]
  [p_a] -> VSG/3(p)
  [q_a_ref] -> VSG/2(q_s_ref)
  p_a_ref/1 -> [p_a_ref]
  q_a_ref/1 -> [q_a_ref]
  p_a/1 -> [p_a]
  q_a/1 -> [q_a]
  [i_sdq_ref_a] -> MATLAB Function3/2(dq)
  [theta_a] -> MATLAB Function3/1(theta)
  Constant2/1 -> MATLAB Function1/1(theta)
  MATLAB Function1/1(dq) -> i_salbe_a_ref/1
  MATLAB Function3/1(abc) -> MATLAB Function1/2(abc)
  [omega_rads_a] -> omega_rads_a/1
  VSG/3(dx) -> Discrete-Time Integrator1/1
  v_salbe_a/1 -> [v_salbe_a]
  [v_salbe_a] -> MATLAB Function2/1(alpha_beta)
  [theta_a] -> MATLAB Function2/2(theta)
  MATLAB Function2/1(dq) -> Unit Delay/1
  [v_sdq_a] -> VSG/6(v_sdq)
  Unit Delay/1 -> Scope1/1, [v_sdq_a]
  Unit Delay1/1 -> [i_sdq_a]
  MATLAB Function4/1(dq) -> Unit Delay1/1
  [theta_a] -> MATLAB Function4/2(theta)
  [i_salbe_a] -> MATLAB Function4/1(alpha_beta)
  i_salbe_a/1 -> [i_salbe_a]
  [i_sdq_a] -> VSG/5(i_sdq)
  [omega_pll] -> Gain/1
  Step1/1 -> Switch/2
  Constant1/1 -> Switch/1
  Gain/1 -> Switch/3
  omega_pll/1 -> [omega_pll]
  Switch/1 -> VSG/8(omega_base)
  Step2/1 -> Discrete-Time Integrator1/2
  First-Order Filter/1 -> Scope2/1, [i_sdq_ref_a]

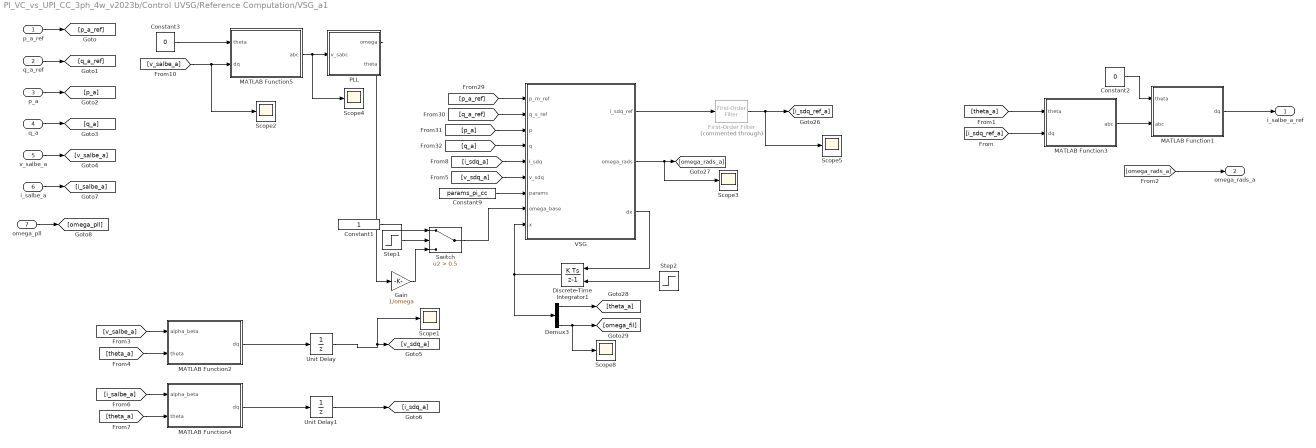
== system PI_VC_vs_UPI_CC_3ph_4w_v2023b/Control UVSG/Reference Computation/VSG_a1 ==
  p_a_ref : Inport
  q_a_ref : Inport  Port=2
  p_a : Inport  Port=3
  q_a : Inport  Port=4
  v_salbe_a : Inport  Port=5
  i_salbe_a : Inport  Port=6
  omega_pll : Inport  Port=7
  Constant1 : Constant
  Constant2 : Constant  Value=0
  Constant3 : Constant  Value=0
  Constant9 : Constant  Value=params_pi_cc
  Demux3 : Demux
  Discrete-Time Integrator1 : DiscreteIntegrator  ExternalReset=rising  InitialCondition=[0;0;0;2*pi*50]  SampleTime=Ts_Control  ICPrevOutput=DiscIntNeverNeededParam  ICPrevScaledInput=DiscIntNeverNeededParam
  First-Order Filter : spsFirstOrderFilterLib/First-Order Filter  Commented=through  FilterType=Lowpass  Tc=2.4e-3  Ts=Ts_Control  Initialize=on  Vac_Init=[0, 0, 60]  Vdc_Init=0  PlotResponse=off  FreqRange="[0,  200,  1]"
  Gain : Gain  Gain=1/omega
  MATLAB Function1 : MATLAB Function  TreatAsAtomicUnit=on
  MATLAB Function2 : MATLAB Function  TreatAsAtomicUnit=on
  MATLAB Function3 : MATLAB Function  TreatAsAtomicUnit=on
  MATLAB Function4 : MATLAB Function  TreatAsAtomicUnit=on
  MATLAB Function5 : MATLAB Function  TreatAsAtomicUnit=on
  PLL : Subsystem
  Scope{1..5,8} (6 alike) : Scope
  Step1 : Step  SampleTime=0
  Step2 : Step  Time=0  SampleTime=0
  Switch : Switch  Criteria=u2 > Threshold  Threshold=0.5  SaturateOnIntegerOverflow=off  InputSameDT=off
  Unit Delay : UnitDelay  SampleTime=-1  HasFrameUpgradeWarning=on
  Unit Delay1 : UnitDelay  SampleTime=-1  HasFrameUpgradeWarning=on
  VSG : MATLAB Function  TreatAsAtomicUnit=on
  i_salbe_a_ref : Outport  VectorParamsAs1DForOutWhenUnconnected=off
  omega_rads_a : Outport  Port=2  VectorParamsAs1DForOutWhenUnconnected=off
  wires:
  First-Order Filter/1 -> Scope5/1, [i_sdq_ref_a]
  Step2/1 -> Discrete-Time Integrator1/2
  Switch/1 -> VSG/8(omega_base)
  omega_pll/1 -> [omega_pll]
  Gain/1 -> Switch/3
  Constant1/1 -> Switch/1
  Step1/1 -> Switch/2
  [i_sdq_a] -> VSG/5(i_sdq)
  i_salbe_a/1 -> [i_salbe_a]
  [i_salbe_a] -> MATLAB Function4/1(alpha_beta)
  [theta_a] -> MATLAB Function4/2(theta)
  MATLAB Function4/1(dq) -> Unit Delay1/1
  Unit Delay1/1 -> [i_sdq_a]
  Unit Delay/1 -> [v_sdq_a], Scope1/1
  [v_sdq_a] -> VSG/6(v_sdq)
  MATLAB Function2/1(dq) -> Unit Delay/1
  [theta_a] -> MATLAB Function2/2(theta)
  [v_salbe_a] -> MATLAB Function2/1(alpha_beta)
  v_salbe_a/1 -> [v_salbe_a]
  VSG/3(dx) -> Discrete-Time Integrator1/1
  [omega_rads_a] -> omega_rads_a/1
  MATLAB Function3/1(abc) -> MATLAB Function1/2(abc)
  MATLAB Function1/1(dq) -> i_salbe_a_ref/1
  Constant2/1 -> MATLAB Function1/1(theta)
  [theta_a] -> MATLAB Function3/1(theta)
  [i_sdq_ref_a] -> MATLAB Function3/2(dq)
  q_a/1 -> [q_a]
  p_a/1 -> [p_a]
  q_a_ref/1 -> [q_a_ref]
  p_a_ref/1 -> [p_a_ref]
  [q_a_ref] -> VSG/2(q_s_ref)
  [p_a] -> VSG/3(p)
  VSG/2(omega_rads) -> [omega_rads_a], Scope3/1
  Discrete-Time Integrator1/1 -> VSG/9(x), Demux3/1
  VSG/1(i_sdq_ref) -> First-Order Filter/1
  Demux3/1 -> [theta_a]
  Demux3/4 -> [omega_fil], Scope8/1
  Constant9/1 -> VSG/7(params)
  [q_a] -> VSG/4(q)
  [p_a_ref] -> VSG/1(p_m_ref)
  MATLAB Function5/1(abc) -> Scope4/1, PLL/1(v_sabc)
  [v_salbe_a] -> Scope2/1, MATLAB Function5/2(dq)
  Constant3/1 -> MATLAB Function5/1(theta)
  PLL/1(omega) -> Gain/1

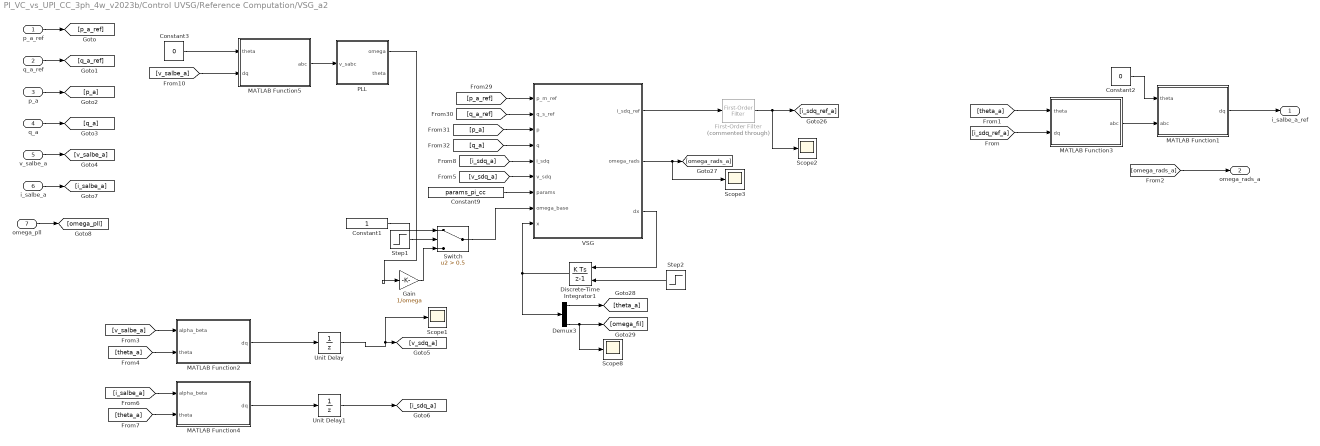
== system PI_VC_vs_UPI_CC_3ph_4w_v2023b/Control UVSG/Reference Computation/VSG_a2 ==
  p_a_ref : Inport
  q_a_ref : Inport  Port=2
  p_a : Inport  Port=3
  q_a : Inport  Port=4
  v_salbe_a : Inport  Port=5
  i_salbe_a : Inport  Port=6
  omega_pll : Inport  Port=7
  Constant1 : Constant
  Constant2 : Constant  Value=0
  Constant3 : Constant  Value=0
  Constant9 : Constant  Value=params_pi_cc
  Demux3 : Demux
  Discrete-Time Integrator1 : DiscreteIntegrator  ExternalReset=rising  InitialCondition=[0;0;0;2*pi*50]  SampleTime=Ts_Control  ICPrevOutput=DiscIntNeverNeededParam  ICPrevScaledInput=DiscIntNeverNeededParam
  First-Order Filter : spsFirstOrderFilterLib/First-Order Filter  Commented=through  FilterType=Lowpass  Tc=2.4e-3  Ts=Ts_Control  Initialize=on  Vac_Init=[0, 0, 60]  Vdc_Init=0  PlotResponse=off  FreqRange="[0,  200,  1]"
  Gain : Gain  Gain=1/omega
  MATLAB Function1 : MATLAB Function  TreatAsAtomicUnit=on
  MATLAB Function2 : MATLAB Function  TreatAsAtomicUnit=on
  MATLAB Function3 : MATLAB Function  TreatAsAtomicUnit=on
  MATLAB Function4 : MATLAB Function  TreatAsAtomicUnit=on
  MATLAB Function5 : MATLAB Function  TreatAsAtomicUnit=on
  PLL : Subsystem
  Scope{1..3,8} (4 alike) : Scope
  Step1 : Step  SampleTime=0
  Step2 : Step  Time=0  SampleTime=0
  Switch : Switch  Criteria=u2 > Threshold  Threshold=0.5  SaturateOnIntegerOverflow=off  InputSameDT=off
  Unit Delay : UnitDelay  SampleTime=-1  HasFrameUpgradeWarning=on
  Unit Delay1 : UnitDelay  SampleTime=-1  HasFrameUpgradeWarning=on
  VSG : MATLAB Function  TreatAsAtomicUnit=on
  i_salbe_a_ref : Outport  VectorParamsAs1DForOutWhenUnconnected=off
  omega_rads_a : Outport  Port=2  VectorParamsAs1DForOutWhenUnconnected=off
  wires:
  [p_a_ref] -> VSG/1(p_m_ref)
  [q_a] -> VSG/4(q)
  Constant9/1 -> VSG/7(params)
  Demux3/4 -> Scope8/1, [omega_fil]
  Demux3/1 -> [theta_a]
  VSG/1(i_sdq_ref) -> First-Order Filter/1
  Discrete-Time Integrator1/1 -> Demux3/1, VSG/9(x)
  VSG/2(omega_rads) -> Scope3/1, [omega_rads_a]
  [p_a] -> VSG/3(p)
  [q_a_ref] -> VSG/2(q_s_ref)
  p_a_ref/1 -> [p_a_ref]
  q_a_ref/1 -> [q_a_ref]
  p_a/1 -> [p_a]
  q_a/1 -> [q_a]
  [i_sdq_ref_a] -> MATLAB Function3/2(dq)
  [theta_a] -> MATLAB Function3/1(theta)
  Constant2/1 -> MATLAB Function1/1(theta)
  MATLAB Function1/1(dq) -> i_salbe_a_ref/1
  MATLAB Function3/1(abc) -> MATLAB Function1/2(abc)
  [omega_rads_a] -> omega_rads_a/1
  VSG/3(dx) -> Discrete-Time Integrator1/1
  v_salbe_a/1 -> [v_salbe_a]
  [v_salbe_a] -> MATLAB Function2/1(alpha_beta)
  [theta_a] -> MATLAB Function2/2(theta)
  MATLAB Function2/1(dq) -> Unit Delay/1
  [v_sdq_a] -> VSG/6(v_sdq)
  Unit Delay/1 -> Scope1/1, [v_sdq_a]
  Unit Delay1/1 -> [i_sdq_a]
  MATLAB Function4/1(dq) -> Unit Delay1/1
  [theta_a] -> MATLAB Function4/2(theta)
  [i_salbe_a] -> MATLAB Function4/1(alpha_beta)
  i_salbe_a/1 -> [i_salbe_a]
  [i_sdq_a] -> VSG/5(i_sdq)
  Step1/1 -> Switch/2
  Constant1/1 -> Switch/1
  Gain/1 -> Switch/3
  omega_pll/1 -> [omega_pll]
  Switch/1 -> VSG/8(omega_base)
  Step2/1 -> Discrete-Time Integrator1/2
  First-Order Filter/1 -> Scope2/1, [i_sdq_ref_a]
  [v_salbe_a] -> MATLAB Function5/2(dq)
  MATLAB Function5/1(abc) -> PLL/1(v_sabc)
  Constant3/1 -> MATLAB Function5/1(theta)
  PLL/1(omega) -> Gain/1

== system PI_VC_vs_UPI_CC_3ph_4w_v2023b/Control UVSG/Control corriente en alpha-beta/Resonant Controller. Double Integrator/Subsystem1 ==
  error : Inport
  omega_PLL : Inport  Port=2
  Discrete-Time Integrator8 : DiscreteIntegrator  SampleTime=-1  ICPrevOutput=DiscIntNeverNeededParam  ICPrevScaledInput=DiscIntNeverNeededParam
  Discrete-Time Integrator9 : DiscreteIntegrator  IntegratorMethod=Integration: Backward Euler  SampleTime=-1  ICPrevOutput=DiscIntNeverNeededParam  ICPrevScaledInput=DiscIntNeverNeededParam
  Kr_a : Gain  Gain=Kr_i
  Product : Product  Inputs=3
  Sum1 : Sum  Inputs=|+-
  "omega_PLL " : InportShadow  Port=2
  out : Outport  VectorParamsAs1DForOutWhenUnconnected=off
  wires:
  "omega_PLL "/1 -> Product/3
  omega_PLL/1 -> Product/2
  Kr_a/1 -> Sum1/1
  Sum1/1 -> Discrete-Time Integrator8/1
  Discrete-Time Integrator8/1 -> out/1, Product/1
  Product/1 -> Discrete-Time Integrator9/1
  error/1 -> Kr_a/1
  Discrete-Time Integrator9/1 -> Sum1/2

== system PI_VC_vs_UPI_CC_3ph_4w_v2023b/Control UVSG/Control corriente en alpha-beta/Resonant Controller. Double Integrator/Subsystem2 ==
  error : Inport
  omega_PLL : Inport  Port=2
  Discrete-Time Integrator8 : DiscreteIntegrator  SampleTime=-1  ICPrevOutput=DiscIntNeverNeededParam  ICPrevScaledInput=DiscIntNeverNeededParam
  Discrete-Time Integrator9 : DiscreteIntegrator  IntegratorMethod=Integration: Backward Euler  SampleTime=-1  ICPrevOutput=DiscIntNeverNeededParam  ICPrevScaledInput=DiscIntNeverNeededParam
  Kr_a : Gain  Gain=Kr_i
  Product : Product  Inputs=3
  Sum1 : Sum  Inputs=|+-
  "omega_PLL " : InportShadow  Port=2
  out : Outport  VectorParamsAs1DForOutWhenUnconnected=off
  wires:
  Discrete-Time Integrator9/1 -> Sum1/2
  error/1 -> Kr_a/1
  Product/1 -> Discrete-Time Integrator9/1
  Discrete-Time Integrator8/1 -> Product/1, out/1
  Sum1/1 -> Discrete-Time Integrator8/1
  Kr_a/1 -> Sum1/1
  omega_PLL/1 -> Product/2
  "omega_PLL "/1 -> Product/3

== system PI_VC_vs_UPI_CC_3ph_4w_v2023b/Control UVSG/Control corriente en alpha-beta/Resonant Controller. Impulse invariant/Subsystem ==
  error : Inport
  omega_PLL : Inport  Port=2
  Gain1 : Gain  Gain=Kr_i
  MATLAB Function : MATLAB Function  TreatAsAtomicUnit=on
  Unit Delay : UnitDelay  SampleTime=Ts_Control  HasFrameUpgradeWarning=on
  Unit Delay1 : UnitDelay  SampleTime=Ts_Control  HasFrameUpgradeWarning=on
  Unit Delay2 : UnitDelay  SampleTime=Ts_Control  HasFrameUpgradeWarning=on
  y : Outport
  wires:
  Unit Delay2/1 -> MATLAB Function/3(u_1)
  MATLAB Function/1(y) -> y/1, Unit Delay/1
  error/1 -> Gain1/1
  omega_PLL/1 -> MATLAB Function/1(omega_vsg)
  Unit Delay/1 -> MATLAB Function/4(y_1), Unit Delay1/1
  Unit Delay1/1 -> MATLAB Function/5(y_2)
  Gain1/1 -> Unit Delay2/1, MATLAB Function/2(u)
